simulink model "feedbacksimplified"  (R2013a)
settings: Solver=ode45  StartTime=0.0  StopTime=20  RelTol=1e-3
values from neighbouring files (symbols this model uses):
  A = [0.8 0.3; 0 -0.6]    [setup.m]
  P = dlyap(A',Q)    [setup.m]
  x0 = [1;-0.5]    [setup.m]
undefined symbols (not defined in the file or in its folder): B, F, G
libraries: simulink x6, utils x3
settings Model: Creator=aeagr  LastModifiedBy=aeagr
settings DataIOCC: SignalLoggingSaveFormat=ModelDataLogs
settings OptimizationCC: ExpressionDepthLimit=2147483647
settings DebuggingCC: MultiTaskDSMMsg=warning  MultiTaskCondExecSysMsg=none  FcnCallInpInsideContextMsg=EnableAllAsWarning  StrictBusMsg=None
settings RTWCC: IncludeERTFirstTime=on

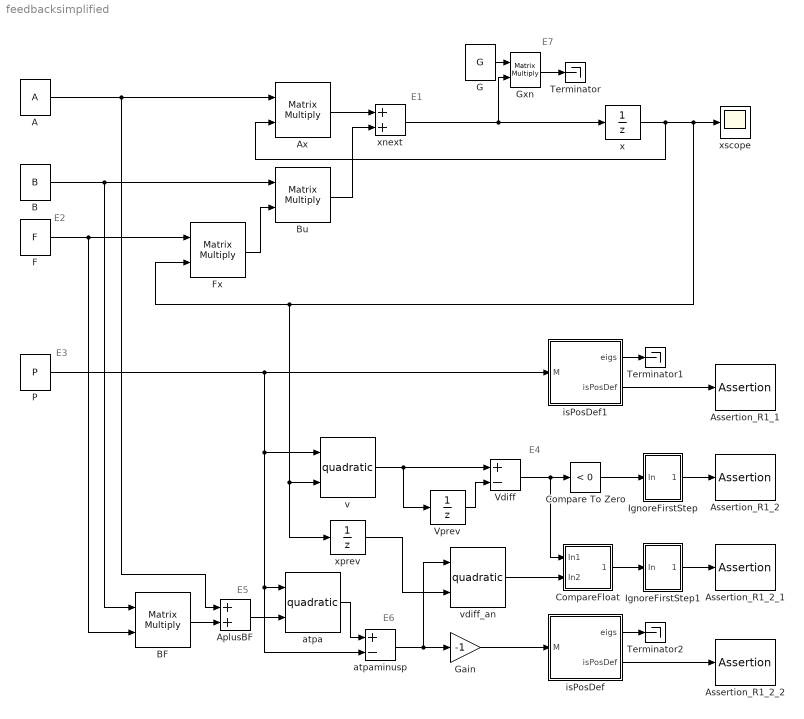
== system feedbacksimplified ==
  note: E7
  note: E6
  note: E5
  note: E4
  note: E3
  note: E2
  note: E1
  A : Constant  Value=A
  AplusBF : Sum
  Assertion_R1_1 : Assertion
  Assertion_R1_2 : Assertion
  Assertion_R1_2_1 : Assertion  Enabled=off
  Assertion_R1_2_2 : Assertion
  Ax : Product  Multiplication=Matrix(*)  RndMeth=Zero
  B : Constant  Value=B
  BF : Product  Multiplication=Matrix(*)  RndMeth=Zero
  Bu : Product  Multiplication=Matrix(*)  RndMeth=Zero
  Compare To Zero : simulink/Logic and Bit Operations/Compare To Zero  relop=<  OutDataTypeStr=boolean
  CompareFloat : Subsystem
  F : Constant  Value=F  VectorParams1D=off
  Fx : Product  Multiplication=Matrix(*)  RndMeth=Zero
  G : Constant  Value=G
  Gain : Gain  Gain=-1
  Gxn : Product  Multiplication=Matrix(*)  RndMeth=Zero
  IgnoreFirstStep : Subsystem  mask(IgnoreFirstStep){}
  IgnoreFirstStep1 : Subsystem  mask(IgnoreFirstStep){}
  P : Constant  Value=P
  Terminator : Terminator
  Terminator1 : Terminator
  Terminator2 : Terminator
  Vdiff : Sum  Inputs=+-  mask(Subtract){}
  Vprev : UnitDelay
  atpa : utils/quadratic  SystemSampleTime=-1
  atpaminusp : Sum  Inputs=+-  mask(Subtract){}
  isPosDef : Subsystem
  isPosDef1 : Subsystem
  v : utils/quadratic  SystemSampleTime=-1
  vdiff_an : utils/quadratic  SystemSampleTime=-1
  x : UnitDelay  InitialCondition=x0
  xnext : Sum
  xprev : UnitDelay  InitialCondition=x0
  xscope : Scope
  wires:
  v/1 -> Vdiff/1, Vprev/1
  Vprev/1 -> Vdiff/2
  IgnoreFirstStep/1(Out) -> Assertion_R1_2/1
  Compare To Zero/1 -> IgnoreFirstStep/1(In)
  atpa/1 -> atpaminusp/1
  vdiff_an/1 -> CompareFloat/2(In2)
  xprev/1 -> vdiff_an/2
  CompareFloat/1(Out1) -> IgnoreFirstStep1/1(In)
  IgnoreFirstStep1/1(Out) -> Assertion_R1_2_1/1
  isPosDef/2(isPosDef) -> Assertion_R1_2_2/1
  Gain/1 -> isPosDef/1(M)
  isPosDef/1(eigs) -> Terminator2/1
  isPosDef1/2(isPosDef) -> Assertion_R1_1/1
  isPosDef1/1(eigs) -> Terminator1/1
  atpaminusp/1 -> vdiff_an/1, Gain/1
  A/1 -> AplusBF/1, Ax/1
  P/1 -> v/1, atpaminusp/2, atpa/1, isPosDef1/1(M)
  Ax/1 -> xnext/1
  Bu/1 -> xnext/2
  B/1 -> BF/1, Bu/1
  Fx/1 -> Bu/2
  x/1 -> Ax/2, Fx/2, v/2, xprev/1, xscope/1
  F/1 -> BF/2, Fx/1
  BF/1 -> AplusBF/2
  AplusBF/1 -> atpa/2
  Vdiff/1 -> CompareFloat/1(In1), Compare To Zero/1
  xnext/1 -> x/1, Gxn/2
  G/1 -> Gxn/1
  Gxn/1 -> Terminator/1

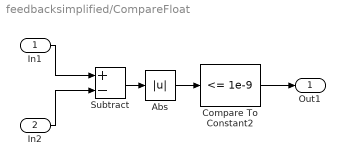
== system feedbacksimplified/CompareFloat ==
  In1 : Inport
  In2 : Inport  Port=2
  Abs : Abs
  Compare To Constant2 : simulink/Logic and Bit Operations/Compare To Constant  relop=<=  const=1e-9  OutDataTypeStr=boolean
  Subtract : Sum  Inputs=+-
  Out1 : Outport
  wires:
  Subtract/1 -> Abs/1
  Abs/1 -> Compare To Constant2/1
  In1/1 -> Subtract/1
  Compare To Constant2/1 -> Out1/1
  In2/1 -> Subtract/2

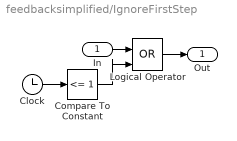
== system feedbacksimplified/IgnoreFirstStep ==
  In : Inport
  Clock : Clock
  Compare To Constant : simulink/Logic and Bit Operations/Compare To Constant  relop=<=  const=1  OutDataTypeStr=boolean
  Logical Operator : Logic  Operator=OR  IconShape=distinctive  AllPortsSameDT=off  OutDataTypeStr=boolean
  Out : Outport
  wires:
  Clock/1 -> Compare To Constant/1
  Compare To Constant/1 -> Logical Operator/2
  In/1 -> Logical Operator/1
  Logical Operator/1 -> Out/1

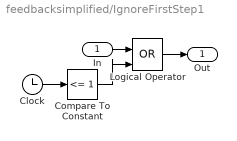
== system feedbacksimplified/IgnoreFirstStep1 ==
  In : Inport
  Clock : Clock
  Compare To Constant : simulink/Logic and Bit Operations/Compare To Constant  relop=<=  const=1  OutDataTypeStr=boolean
  Logical Operator : Logic  Operator=OR  IconShape=distinctive  AllPortsSameDT=off  OutDataTypeStr=boolean
  Out : Outport
  wires:
  Logical Operator/1 -> Out/1
  In/1 -> Logical Operator/1
  Compare To Constant/1 -> Logical Operator/2
  Clock/1 -> Compare To Constant/1

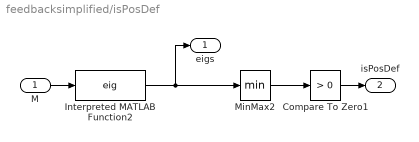
== system feedbacksimplified/isPosDef ==
  M : Inport
  Compare To Zero1 : simulink/Logic and Bit Operations/Compare To Zero  relop=>  OutDataTypeStr=boolean
  Interpreted MATLAB Function2 : MATLABFcn  MATLABFcn=eig
  MinMax2 : MinMax
  eigs : Outport
  isPosDef : Outport  Port=2
  wires:
  MinMax2/1 -> Compare To Zero1/1
  Interpreted MATLAB Function2/1 -> MinMax2/1, eigs/1
  Compare To Zero1/1 -> isPosDef/1
  M/1 -> Interpreted MATLAB Function2/1

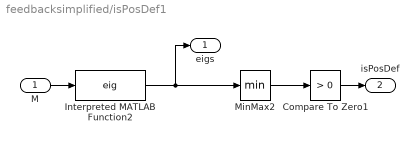
== system feedbacksimplified/isPosDef1 ==
  M : Inport
  Compare To Zero1 : simulink/Logic and Bit Operations/Compare To Zero  relop=>  OutDataTypeStr=boolean
  Interpreted MATLAB Function2 : MATLABFcn  MATLABFcn=eig
  MinMax2 : MinMax
  eigs : Outport
  isPosDef : Outport  Port=2
  wires:
  M/1 -> Interpreted MATLAB Function2/1
  Compare To Zero1/1 -> isPosDef/1
  Interpreted MATLAB Function2/1 -> eigs/1, MinMax2/1
  MinMax2/1 -> Compare To Zero1/1
